simulink model "four_tanks_1_1_resilient"  (R2017a)
settings: Solver=ode45  StartTime=0.0  StopTime=150  RelTol=1e-3  EnableMultiTasking=on
model workspace (MATLAB code in the model file):
  | alpha = 32; % tank cross sectional area (cm^2)
  | gamma1 = 0.7; % inlet valve coefficient 1
  | gamma2 = 0.5; % inlet valve coefficient 2
  | k = 5; % pump coefficient (cm^3/Vs)
  | a = 4; % outlet valve coefficient
  | x0 = 0; % init level difference
  | 
  | h0 = 1.5625; % init level
  | 
  | Ts = 1;
settings Model: ExtModeAutoUpdateStatusClock=off  Creator=arun  LastModifiedBy=michelbarbeau
settings DataIOCC: SaveFormat=Array  SignalLoggingSaveFormat=ModelDataLogs  SaveState=on
settings OptimizationCC: ExpressionDepthLimit=2147483647  InitFltsAndDblsToZero=on  LifeSpan=inf
settings DebuggingCC: SaveWithParameterizedLinksMsg=none  UnderspecifiedInitializationDetection=Classic  MergeDetectMultiDrivingBlocksExec=none  SolverPrmCheckMsg=warning  FcnCallInpInsideContextMsg=warning  StateNameClashWarn=warning  SFUnexpectedBacktrackingDiag=warning  SFNoUnconditionalDefaultTransitionDiag=warning  SFExecutionAtInitializationDiag=none
settings HardwareCC: ProdBitPerPointer=32  ProdBitPerSizeT=32  ProdBitPerPtrDiffT=32  ProdLargestAtomicFloat=None  ProdIntDivRoundTo=Undefined  ProdEndianess=Unspecified  ProdWordSize=32  ProdHWDeviceType=32-bit Generic
settings ModelReferenceCC: PropagateSignalLabelsOutOfModel=off
settings GRTTargetCC: TargetFcnLib=ansi_tfl_tmw.mat  TargetLangStandard=C89/C90 (ANSI)  GeneratePreprocessorConditionals=Disable all  CombineOutputUpdateFcns=off  GRTInterface=on
settings ConfigComp: CovMetricSettings=dw  CovHtmlReporting=on  CovSaveCumulativeToWorkspaceVar=on  CovSaveSingleToWorkspaceVar=on  CovExternalEMLEnable=off

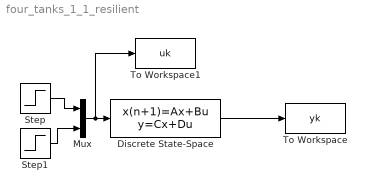
== system four_tanks_1_1_resilient ==
  Discrete State-Space : DiscreteStateSpace  A="[ -a/( alpha*2*sqrt(h0) ) 0 a/( alpha*2*sqrt(h0) )  0;0   -a/( alpha*2*sqrt(h0) ) 0 a/( alpha*2*sqrt(h0) ) ; 0   0 -a/( alpha*2*sqrt(h0) ) 0  ; 0   0 0 -a/( alpha*2*sqrt(h0) ) ]"  B=[ gamma1*k/alpha 0; 0 gamma2*k/alpha; 1-gamma1*k/alpha 0; 0 1-gamma2*k/alpha; ]  C=[ 1 0 0 0; 0 1 0 0; 0 0 1 0; 0 0 0 1 ]  D=[0 0; 0 0; 0 0; 0 0]  SampleTime=-1
  Mux : Mux  Inputs=2
  Step : Step  Before=1  SampleTime=0
  Step1 : Step  Before=0.8  After=0.8  SampleTime=0
  To Workspace : ToWorkspace  VariableName=yk  SampleTime=Ts
  To Workspace1 : ToWorkspace  VariableName=uk  SampleTime=Ts
  wires:
  Discrete State-Space/1 -> To Workspace/1
  Step1/1 -> Mux/2
  Mux/1 -> To Workspace1/1, Discrete State-Space/1
  Step/1 -> Mux/1
